simulink model "RL_fault_tolerance_simulation"  (R2024b)
settings: Solver=FixedStepAuto  StartTime=0.0  StopTime=500  FixedStep=0.1  RelTol=1e-3
PostLoadFcn:
  | RL_fault_tolerance_Setup
values from neighbouring files (symbols this model uses):
  D_default = 10    [rl_tolernace.m]
  t_gap = 1.4    [rl_tolernace.m]
  Ts = 0.1    [rl_tolernace.m]
  v_set = 28    [rl_tolernace.m]
undefined symbols (not defined in the file or in its folder): DiscIntNeverNeededParam, driving, egoID, lr, m, matlabshared, posSelector, R, tau
libraries: simulink x5, drivingscenarioandsensors x3, drivinglib x2, trackingutilitieslib x1, rllib x1, autolibshared x1
settings Model: SnapshotInterval=5  Creator=The MathWorks, Inc.  LastModifiedBy=user
settings SolverCC: AlgebraicLoopSolver=TrustRegion  MinimalZcImpactIntegration=on
settings OptimizationCC: DefaultParameterBehavior=Inlined  InlineInvariantSignals=on  ReuseModelBlockBuffer=off  PassReuseOutputArgsAs=Individual arguments  ZeroExternalMemoryAtStartup=off  OptimizeBlockOrder=speed  EfficientTunableParamExpr=on
settings DebuggingCC: ParameterTunabilityLossMsg=error  UnconnectedInputMsg=warning  UnconnectedOutputMsg=warning  UnconnectedLineMsg=warning  PregeneratedLibrarySubsystemCodeDiagnostic=none  ArithmeticOperatorsInVariantConditions=warning
settings HardwareCC: ProdLongLongMode=on
settings ModelReferenceCC: EnableRefExpFcnMdlSchedulingChecks=on  ModelReferenceNumInstancesAllowed=Single  PropagateVarSize=Only when enabling
settings SFSimCC: SimUseLocalCustomCode=off  CustomCodeUndefinedFunction=UseInterfaceOnly
settings RTWCC: Description=Embedded Coder  SystemTargetFile=ert.tlc  TemplateMakefile=ert_default_tmf  GenerateReport=on  RTWUseLocalCustomCode=off  BuildConfiguration=Faster Runs  IncludeHyperlinkInReport=on  LaunchReport=on  GenerateTraceInfo=on  GenerateTraceReport=on  GenerateTraceReportSl=on  GenerateTraceReportSf=on  GenerateTraceReportEml=on  GenerateCodeMetricsReport=on  GPUComputeCapability=3.5  DLArmComputeVersion=19.05
settings CodeAppCC: ForceParamTrailComments=on  IgnoreCustomStorageClasses=off  OperatorAnnotations=on  SimulinkDataObjDesc=on  SFDataObjDesc=on  CustomSymbolStrFcn=$N$M$F  InsertBlockDesc=on
settings ERTTargetCC: TargetLangStandard=C99 (ISO)  GenerateSampleERTMain=on  CombineSignalStateStructs=on  SuppressErrorStatus=on  RootIOFormat=Structure reference  RTWCAPISignals=on  ERTCustomFileTemplate=example_file_process.tlc  DynamicArrayContainerType=coder::array

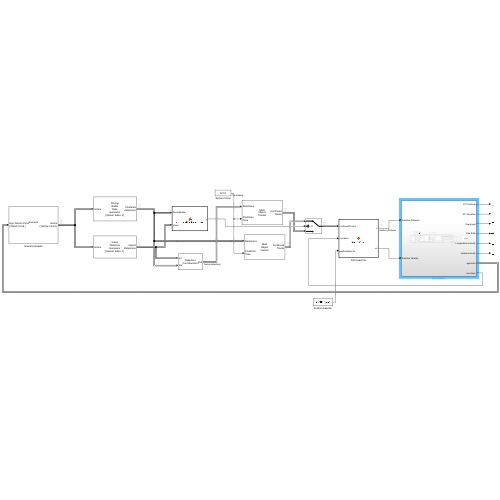
[thumbnail: Simulink's stored preview of the top-level diagram]
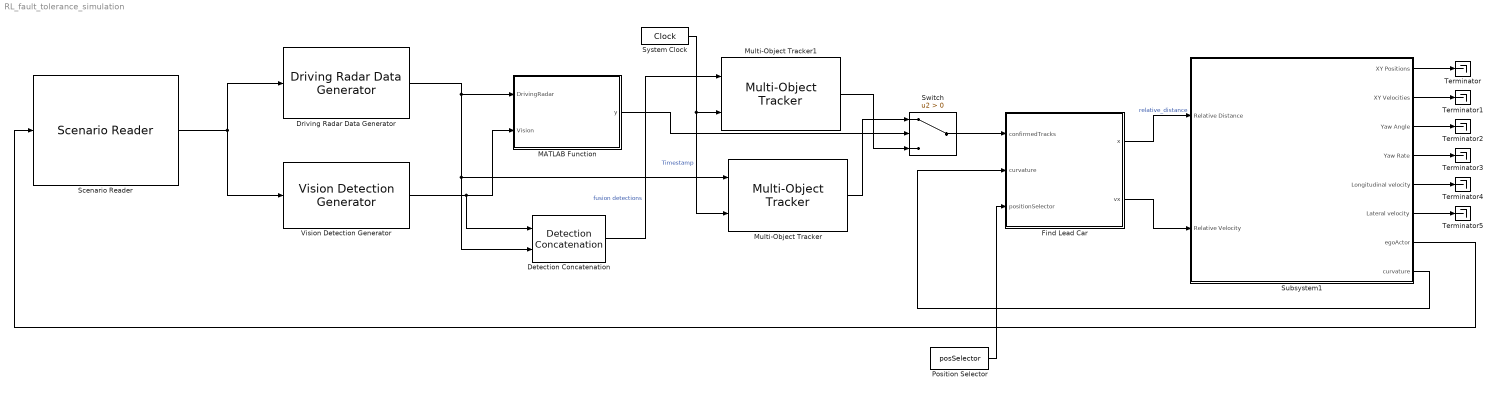
== system RL_fault_tolerance_simulation ==
  Detection Concatenation : trackingutilitieslib/Detection Concatenation  NumInputs=2  BusNameSource=Property  BusName=BusDetectionConcatenation  SimulateUsing=Interpreted execution
  Driving Radar Data Generator : drivingscenarioandsensors/Driving Radar Data Generator  SensorIndex=2  UpdateRate=10  MountingLocation=[ 3.7, 0, 0.2 ]  MountingAngles=[0 0 0]  HasElevation=off  HasRangeRate=on  HasNoise=on  HasFalseAlarms=on  HasOcclusion=on  MaxNumReportsSource=Property  MaxNumReports=50  TargetReportFormat=Clustered detections  DetectionCoordinates=Body  TrackCoordinates=Body  BusNameSource=Property  BusName=BusRadar  SimulateUsing=Interpreted execution  AzimuthResolution=4  ElevationResolution=5  RangeResolution=2.5  RangeRateResolution=0.5  AzimuthBiasFraction=0.1  ElevationBiasFraction=0.1  RangeBiasFraction=0.05  RangeRateBiasFraction=0.05  FieldOfView=[ 20, 5 ]  RangeLimits=[ 0, 174 ]  RangeRateLimits=[ -100, 100 ]  DetectionProbability=0.9  FalseAlarmRate=1e-06  ReferenceRange=100  ReferenceRCS=0  CenterFrequency=77e9  FilterInitializationFcn=initcvekf  ConfirmationThreshold=[2 3]  DeletionThreshold=[5 5]  InitialSeedSource=Repeatable  InitialSeed=0  UsedSeed=matlabshared.tracking.internal.SimulinkUtilities.seedManager(gcb)  ProfilesSource=Parameters  ProfilesParameters=driving.internal.ActorProfilesRadarParameters  ProfilesExpression=struct('ClassID',0,'Length',4.7,'Width',1.8,'Height',1.4,'OriginOffset',[-1.35 0 0],'RCSPattern',[10 10;10 10],'RCSAzimuthAngles',[-180 180],'RCSElevationAngles',[-90 90])
  Find Lead Car : MATLAB Function  TreatAsAtomicUnit=on
  MATLAB Function : MATLAB Function  TreatAsAtomicUnit=on
  Multi-Object Tracker : drivinglib/Multi-Object Tracker  TrackerIndex=uint32( 0 )  FilterInitializationFcn=initcvekf  AssignmentThreshold=assigThresh  ConfirmationThreshold=[ 2, 3 ]  DeletionThreshold=[ 5, 5 ]  MaxNumTracks=numTracks  MaxNumSensors=numSensors  OOSMHandling=Terminate  StateParametersSimulink=struct  HasStateParametersInput=off  TimeInputSource=Input port  HasCostMatrixInput=off  HasDetectableTrackIDsInput=off  BusNameSource=Property  BusName=BusMultiObjectTracker  TentativeTracksOutputPort=off  AllTracksOutputPort=off  SimulateUsing=Interpreted execution
  Multi-Object Tracker1 : drivinglib/Multi-Object Tracker  TrackerIndex=uint32( 0 )  FilterInitializationFcn=initcvekf  AssignmentThreshold=assigThresh  ConfirmationThreshold=[ 2, 3 ]  DeletionThreshold=[ 5, 5 ]  MaxNumTracks=numTracks  MaxNumSensors=numSensors  OOSMHandling=Terminate  StateParametersSimulink=struct  HasStateParametersInput=off  TimeInputSource=Input port  HasCostMatrixInput=off  HasDetectableTrackIDsInput=off  BusNameSource=Property  BusName=BusMultiObjectTracker  TentativeTracksOutputPort=off  AllTracksOutputPort=off  SimulateUsing=Interpreted execution
  Position Selector : Constant  Value=posSelector
  Scenario Reader : drivingscenarioandsensors/Scenario Reader  ScenarioSource=From workspace  ScenarioFileName=ACCTestBenchScenario.mat  ScenarioVariableName=scenario  OutputCoordinateSystem=Vehicle coordinates  EgoVehicleSource=Input port  EgoVehicleActorID=egoID  OrientVehiclesOnRoad=off  OutputEgoVehiclePose=off  OutputEgoVehicleState=off  SampleTime=0.1  LaneBoundaryOutput=None  LaneBoundaryDistance=0:0.5:9.5  LaneBoundaryLocation=Center of lane markings  BusNameSource=Property  BusName=BusActors  BusNumActorsSource=Scenario  BusNumActors=100  BusName2Source=Auto  BusName2=BusLaneBoundaries  BusNumLaneBoundariesSource=Scenario  BusNumLaneBoundaries=10  BusName3Source=Auto  BusName3=BusEgoActor  BusName4Source=Auto  BusName4=BusEgoState  ShowCoordinateLabels=on  SimulateUsing=Interpreted execution
  Subsystem1 : Subsystem
  Switch : Switch  Criteria=u2 > Threshold  SaturateOnIntegerOverflow=off  InputSameDT=off
  System Clock : DigitalClock  SampleTime=Ts
  Terminator{,1..5} (6 alike) : Terminator
  Vision Detection Generator : drivingscenarioandsensors/Vision Detection Generator  SensorIndex=1  DetectorOutput=Objects only  UpdateInterval=0.1  LaneUpdateInterval=0.1  SensorLocation=[ 2.1, 0 ]  Height=1.1  Yaw=0  Pitch=1  Roll=0  BusNameSource=Property  BusName=BusVision  BusName2Source=Auto  BusName2=BusLaneDetections  MaxNumDetectionsSource=Property  MaxNumDetections=20  MaxNumLanesSource=Property  MaxNumLanes=30  DetectionCoordinates=Ego Cartesian  SimulateUsing=Interpreted execution  MaxRange=150  BoundingBoxAccuracy=5  ProcessNoiseIntensity=5  MaxSpeed=50  MaxAllowedOcclusion=0.5  MinObjectImageSize=[ 15, 15 ]  DetectionProbability=0.9  FalsePositivesPerImage=0.1  MinLaneImageSize=[ 20, 5 ]  LaneBoundaryAccuracy=3  HasNoise=on  InitialSeedSource=Repeatable  InitialSeed=0  UsedSeed=driving.internal.SimulinkUtilities.seedManager(gcb)  ActorProfilesSource=Parameters  ActorProfilesParameters=driving.internal.ActorProfilesParameters  ActorProfilesExpression=struct( 'ClassID', 0, 'Length', 4.7, 'Width', 1.8, 'Height', 1.4, 'OriginOffset', [ -1.35, 0, 0 ] )  Intrinsics=driving.internal.cameraIntrinsics
  wires:
  Subsystem1/1(XY Positions) -> Terminator/1
  Subsystem1/2(XY Velocities) -> Terminator1/1
  Subsystem1/3(Yaw Angle) -> Terminator2/1
  Subsystem1/4(Yaw Rate) -> Terminator3/1
  Subsystem1/5(Longitudinal velocity) -> Terminator4/1
  Subsystem1/6(Lateral velocity) -> Terminator5/1
  Find Lead Car/2(vx) -> Subsystem1/2(Relative Velocity)
  Find Lead Car/1(x) -> Subsystem1/1(Relative Distance)  "relative_distance"
  Subsystem1/8(curvature) -> Find Lead Car/2(curvature)
  Multi-Object Tracker/1 -> Switch/1
  System Clock/1 -> Multi-Object Tracker1/2, Multi-Object Tracker/2  "Timestamp"
  Position Selector/1 -> Find Lead Car/3(positionSelector)
  Subsystem1/7(egoActor) -> Scenario Reader/1
  Detection Concatenation/1 -> Multi-Object Tracker1/1  "fusion detections"
  Switch/1 -> Find Lead Car/1(confirmedTracks)
  Driving Radar Data Generator/1 -> Multi-Object Tracker/1, Detection Concatenation/2, MATLAB Function/1(DrivingRadar)
  Scenario Reader/1 -> Driving Radar Data Generator/1, Vision Detection Generator/1
  Vision Detection Generator/1 -> MATLAB Function/2(Vision), Detection Concatenation/1
  MATLAB Function/1(y) -> Switch/2
  Multi-Object Tracker1/1 -> Switch/3

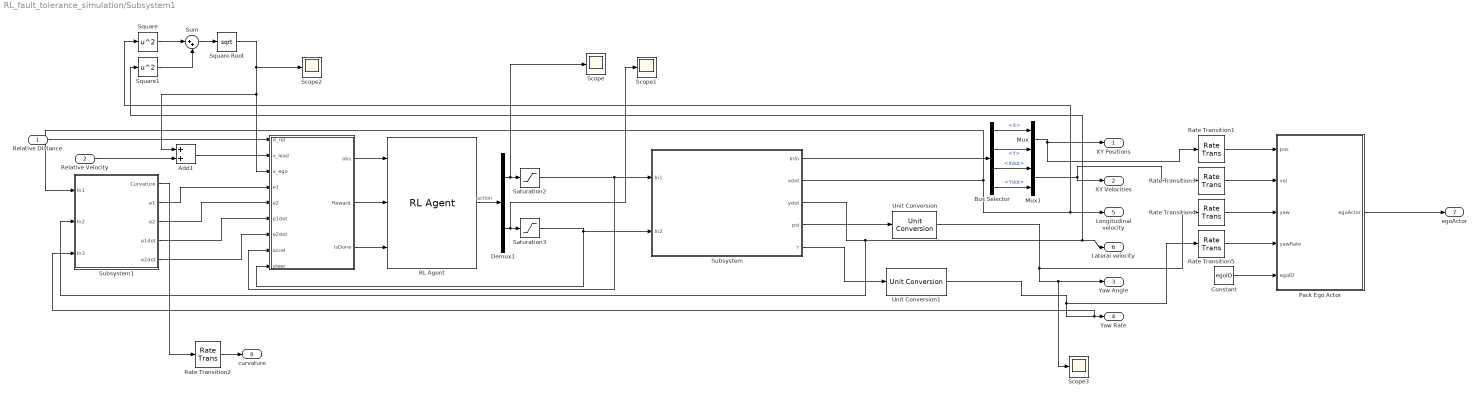
== system RL_fault_tolerance_simulation/Subsystem1 ==
  Relative Distance : Inport
  Relative Velocity : Inport  Port=2
  " " : Subsystem
  Add1 : Sum
  Bus Selector : BusSelector  OutputSignals=InertFrm.FrntAxl.Disp.X,InertFrm.FrntAxl.Disp.Y,InertFrm.FrntAxl.Vel.Xdot,InertFrm.FrntAxl.Vel.Ydot
  Constant : Constant  Value=egoID
  Demux1 : Demux  Outputs=2
  Mux : Mux  Inputs=2
  Mux1 : Mux  Inputs=2
  Pack Ego Actor : MATLAB Function  TreatAsAtomicUnit=on
  RL Agent : rllib/RL Agent  Agent=agent  ExternalActionAsInput=off  ProvideLastAction=off  ProvideCumRwd=off  TreatAsDirectFeedthrough=on  UseStrictObservationDataTypes=off
  Rate Transition{1..5} (5 alike) : RateTransition  OutPortSampleTime=Ts
  Saturation2 : Saturate  UpperLimit=2  LowerLimit=-3
  Saturation3 : Saturate  UpperLimit=0.1  LowerLimit=-0.1
  Scope{,1..3} (4 alike) : Scope
  Square : Math  Operator=square
  Square Root : Sqrt
  Square1 : Math  Operator=square
  Subsystem : Subsystem
  Subsystem1 : Subsystem
  Sum : Sum  Inputs=|++
  Unit Conversion : UnitConversion
  Unit Conversion1 : UnitConversion
  XY Positions : Outport  Unit=m  VectorParamsAs1DForOutWhenUnconnected=off
  XY Velocities : Outport  Port=2  Unit=m/s  VectorParamsAs1DForOutWhenUnconnected=off
  Yaw Angle : Outport  Port=3  Unit=deg  VectorParamsAs1DForOutWhenUnconnected=off
  Yaw Rate : Outport  Port=4  Unit=degree/s  VectorParamsAs1DForOutWhenUnconnected=off
  Longitudinal velocity : Outport  Port=5  VectorParamsAs1DForOutWhenUnconnected=off
  Lateral velocity : Outport  Port=6  VectorParamsAs1DForOutWhenUnconnected=off
  egoActor : Outport  Port=7
  curvature : Outport  Port=8
  wires:
  Bus Selector/4 -> Mux1/2  "<Ydot>"
  Mux1/1 -> XY Velocities/1, Rate Transition3/1
  Rate Transition2/1 -> curvature/1
  Saturation3/1 -> " "/9(steer), Subsystem/2(In2)
  " "/3(isDone) -> RL Agent/3
  Pack Ego Actor/1(egoActor) -> egoActor/1
  Mux/1 -> Rate Transition1/1, XY Positions/1
  " "/1(obs) -> RL Agent/1
  Constant/1 -> Pack Ego Actor/5(egoID)
  Saturation2/1 -> Subsystem/1(In1), " "/8(accel)
  Demux1/2 -> Scope1/1, Saturation3/1
  Unit Conversion1/1 -> Subsystem1/3(In3), Yaw Rate/1, Rate Transition5/1
  Relative Velocity/1 -> Add1/2
  Demux1/1 -> Scope/1, Saturation2/1
  Bus Selector/3 -> Mux1/1  "<Xdot>"
  Relative Distance/1 -> " "/1(d_rel)
  Rate Transition3/1 -> Pack Ego Actor/2(vel)
  Rate Transition5/1 -> Pack Ego Actor/4(yawRate)
  Rate Transition4/1 -> Pack Ego Actor/3(yaw)
  " "/2(Reward) -> RL Agent/2
  Rate Transition1/1 -> Pack Ego Actor/1(pos)
  Add1/1 -> " "/2(v_lead)
  Bus Selector/2 -> Mux/2  "<Y>"
  Bus Selector/1 -> Mux/1  "<X>"
  Unit Conversion/1 -> Scope3/1, Yaw Angle/1, Rate Transition4/1
  RL Agent/1 -> Demux1/1  "action"
  Subsystem/3(ydot) -> Lateral velocity/1, Square1/1, Subsystem1/2(In2)
  Subsystem/2(xdot) -> Longitudinal velocity/1, Square/1, Subsystem1/1(In1)
  Subsystem/1(Info) -> Bus Selector/1
  Subsystem/4(psi) -> Unit Conversion/1
  Subsystem/5(r) -> Unit Conversion1/1
  Subsystem1/1(Curvature) -> Rate Transition2/1
  Subsystem1/2(e1) -> " "/4(e1)
  Subsystem1/3(e2) -> " "/5(e2)
  Subsystem1/4(e1dot) -> " "/6(e1dot)
  Subsystem1/5(e2dot) -> " "/7(e2dot)
  Square/1 -> Sum/1
  Square1/1 -> Sum/2
  Sum/1 -> Square Root/1
  Square Root/1 -> " "/3(v_ego), Add1/1, Scope2/1

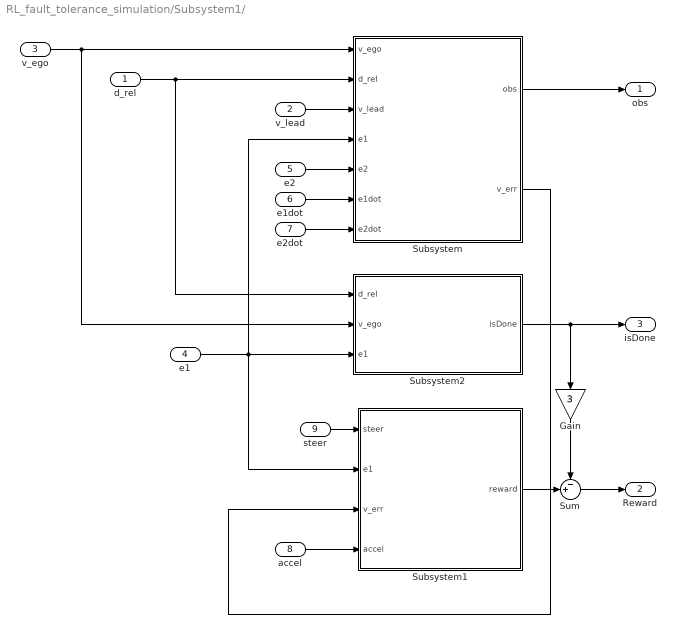
== system RL_fault_tolerance_simulation/Subsystem1/  ==
  d_rel : Inport
  v_lead : Inport  Port=2
  v_ego : Inport  Port=3
  e1 : Inport  Port=4
  e2 : Inport  Port=5
  e1dot : Inport  Port=6
  e2dot : Inport  Port=7
  accel : Inport  Port=8
  steer : Inport  Port=9
  Gain : Gain  Gain=3
  Subsystem : Subsystem
  Subsystem1 : Subsystem
  Subsystem2 : Subsystem
  Sum : Sum  Inputs=-+|
  obs : Outport  VectorParamsAs1DForOutWhenUnconnected=off
  Reward : Outport  Port=2  VectorParamsAs1DForOutWhenUnconnected=off
  isDone : Outport  Port=3  VectorParamsAs1DForOutWhenUnconnected=off
  wires:
  e2dot/1 -> Subsystem/7(e2dot)
  e1/1 -> Subsystem/4(e1), Subsystem2/3(e1), Subsystem1/2(e1)
  e2/1 -> Subsystem/5(e2)
  v_ego/1 -> Subsystem2/2(v_ego), Subsystem/1(v_ego)
  accel/1 -> Subsystem1/4(accel)
  Subsystem2/1(isDone) -> isDone/1, Gain/1
  Subsystem/2(v_err) -> Subsystem1/3(v_err)
  v_lead/1 -> Subsystem/3(v_lead)
  d_rel/1 -> Subsystem2/1(d_rel), Subsystem/2(d_rel)
  steer/1 -> Subsystem1/1(steer)
  Subsystem/1(obs) -> obs/1
  e1dot/1 -> Subsystem/6(e1dot)
  Subsystem1/1(reward) -> Sum/2
  Sum/1 -> Reward/1
  Gain/1 -> Sum/1

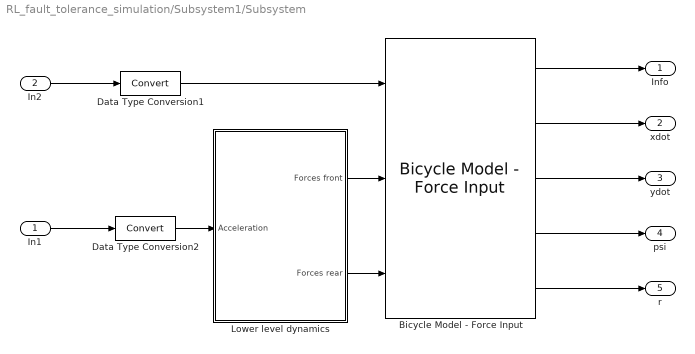
== system RL_fault_tolerance_simulation/Subsystem1/Subsystem ==
  In1 : Inport
  In2 : Inport  Port=2
  Bicycle Model - Force Input : autolibshared/Bicycle Model - Force Input  trackMode=Single (bicycle)  inputMode=External longitudinal forces  frontSteerMode=on  rearSteerMode=off  windMode=off  muMode=off  extFMode=off  extMMode=off  aMode=3  NF=2  NR=2  m=m  a=lf  b=lr  h=0.35  X_o=x0_ego  xdot_o=v0_ego  CalphaMode=off  sigmaMode=on  w=[1.4,1.4]  Cy_f=Cf  Cy_r=Cr  sigma_f=.1  sigma_r=.1  alpha_f_brk=[-.1 .1]  Cy_f_data=[-9e3 9e3]  alpha_r_brk=[-.1 .1]  Cy_r_data=[-9e3 9e3]  Y_o=y0_ego  ydot_o=0  Izz=Iz  psi_o=0  r_o=0  Af=0  Cd=.3  Cl=.1  Cpm=.1  beta_w=[0:0.01:0.3]  Cs=[0:0.03:0.9]  Cym=[0:0.01:0.3]  Pabs=101325  Tair=273  g=9.81  mu=1  xdot_tol=.01  Fznom=5000  Fxtire_sat=1e6  Fytire_sat=1e6  longOff=0  latOff=0  vertOff=0
      settings: LibrarySourceBlock=drivingscenarioandsensors/Bicycle Model - Force Input
  Data Type Conversion1 : DataTypeConversion  SaturateOnIntegerOverflow=off  RndMeth=Floor
  Data Type Conversion2 : DataTypeConversion  SaturateOnIntegerOverflow=off  RndMeth=Floor
  Lower level dynamics : Subsystem
  Info : Outport
  xdot : Outport  Port=2
  ydot : Outport  Port=3
  psi : Outport  Port=4
  r : Outport  Port=5
  wires:
  In1/1 -> Data Type Conversion2/1
  Bicycle Model - Force Input/3 -> ydot/1
  Lower level dynamics/2(Forces rear) -> Bicycle Model - Force Input/3
  Data Type Conversion1/1 -> Bicycle Model - Force Input/1
  Data Type Conversion2/1 -> Lower level dynamics/1(Acceleration)
  Lower level dynamics/1(Forces front) -> Bicycle Model - Force Input/2
  Bicycle Model - Force Input/4 -> psi/1
  Bicycle Model - Force Input/1 -> Info/1
  In2/1 -> Data Type Conversion1/1
  Bicycle Model - Force Input/2 -> xdot/1
  Bicycle Model - Force Input/5 -> r/1

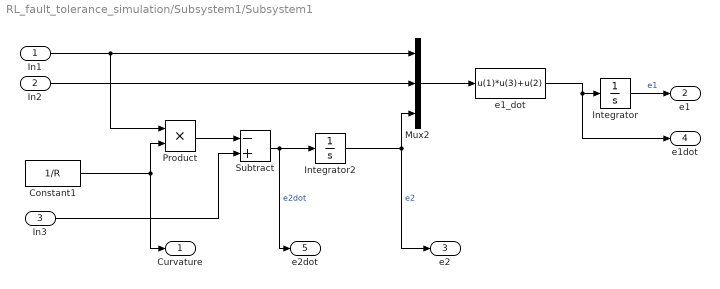
== system RL_fault_tolerance_simulation/Subsystem1/Subsystem1 ==
  In1 : Inport
  In2 : Inport  Port=2
  In3 : Inport  Port=3
  Constant1 : Constant  Value=1/R
  Integrator : Integrator  InitialCondition=0.2
  Integrator2 : Integrator  InitialCondition=-0.1
  Mux2 : Mux  Inputs=[1 1 1]
  Product : Product
  Subtract : Sum  Inputs=-+
  e1_dot : Fcn  Expr=u(1)*u(3)+u(2)
  Curvature : Outport
  e1 : Outport  Port=2
  e2 : Outport  Port=3
  e1dot : Outport  Port=4
  e2dot : Outport  Port=5
  wires:
  Integrator/1 -> e1/1  "e1"
  Constant1/1 -> Product/2, Curvature/1
  Product/1 -> Subtract/1
  In2/1 -> Mux2/2
  In1/1 -> Mux2/1, Product/1
  e1_dot/1 -> e1dot/1, Integrator/1
  Subtract/1 -> Integrator2/1, e2dot/1  "e2dot"
  Integrator2/1 -> e2/1, Mux2/3  "e2"
  Mux2/1 -> e1_dot/1
  In3/1 -> Subtract/2

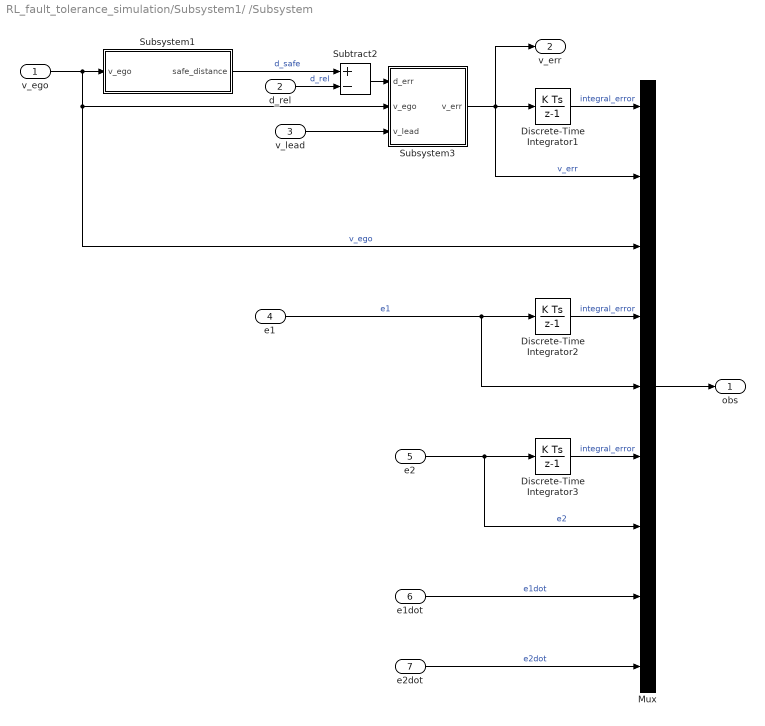
== system RL_fault_tolerance_simulation/Subsystem1/ /Subsystem ==
  v_ego : Inport
  d_rel : Inport  Port=2
  v_lead : Inport  Port=3
  e1 : Inport  Port=4
  e2 : Inport  Port=5
  e1dot : Inport  Port=6
  e2dot : Inport  Port=7
  Discrete-Time Integrator1 : DiscreteIntegrator  SampleTime=-1  ICPrevOutput=DiscIntNeverNeededParam  ICPrevScaledInput=DiscIntNeverNeededParam
  Discrete-Time Integrator2 : DiscreteIntegrator  SampleTime=-1  ICPrevOutput=DiscIntNeverNeededParam  ICPrevScaledInput=DiscIntNeverNeededParam
  Discrete-Time Integrator3 : DiscreteIntegrator  SampleTime=-1  ICPrevOutput=DiscIntNeverNeededParam  ICPrevScaledInput=DiscIntNeverNeededParam
  Mux : Mux  Inputs=9
  Subsystem1 : Subsystem
  Subsystem3 : Subsystem
  Subtract2 : Sum  Inputs=+-
  obs : Outport  VectorParamsAs1DForOutWhenUnconnected=off
  v_err : Outport  Port=2  VectorParamsAs1DForOutWhenUnconnected=off
  wires:
  v_lead/1 -> Subsystem3/3(v_lead)
  Subsystem3/1(v_err) -> v_err/1, Mux/2, Discrete-Time Integrator1/1  "v_err"
  Discrete-Time Integrator3/1 -> Mux/6  "integral_error"
  v_ego/1 -> Mux/3, Subsystem3/2(v_ego), Subsystem1/1(v_ego)  "v_ego"
  d_rel/1 -> Subtract2/2  "d_rel"
  e1/1 -> Mux/5, Discrete-Time Integrator2/1  "e1"
  Subsystem1/1(safe_distance) -> Subtract2/1  "d_safe"
  Discrete-Time Integrator1/1 -> Mux/1  "integral_error"
  e2/1 -> Mux/7, Discrete-Time Integrator3/1  "e2"
  Discrete-Time Integrator2/1 -> Mux/4  "integral_error"
  Mux/1 -> obs/1
  e1dot/1 -> Mux/8  "e1dot"
  e2dot/1 -> Mux/9  "e2dot"
  Subtract2/1 -> Subsystem3/1(d_err)

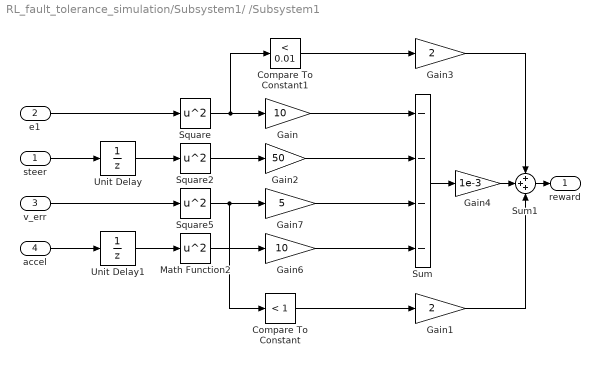
== system RL_fault_tolerance_simulation/Subsystem1/ /Subsystem1 ==
  steer : Inport
  e1 : Inport  Port=2
  v_err : Inport  Port=3
  accel : Inport  Port=4
  Compare To Constant : simulink/Logic and Bit Operations/Compare To Constant  relop=<  const=1  OutDataTypeStr=boolean
  Compare To Constant1 : simulink/Logic and Bit Operations/Compare To Constant  relop=<  const=0.01  OutDataTypeStr=boolean
  Gain : Gain  Gain=10
  Gain1 : Gain  Gain=2
  Gain2 : Gain  Gain=50
  Gain3 : Gain  Gain=2
  Gain4 : Gain  Gain=1e-3
  Gain6 : Gain  Gain=10
  Gain7 : Gain  Gain=5
  Math Function2 : Math  Operator=square  SignedPower=on
  Square : Math  Operator=square  SignedPower=on
  Square2 : Math  Operator=square  SignedPower=on
  Square5 : Math  Operator=square  SignedPower=on
  Sum : Sum  Inputs=----
  Sum1 : Sum  Inputs=+++
  Unit Delay : UnitDelay  SampleTime=-1  HasFrameUpgradeWarning=on
  Unit Delay1 : UnitDelay  SampleTime=-1  HasFrameUpgradeWarning=on
  reward : Outport  VectorParamsAs1DForOutWhenUnconnected=off
  wires:
  e1/1 -> Square/1
  Gain/1 -> Sum/1
  Square/1 -> Compare To Constant1/1, Gain/1
  steer/1 -> Unit Delay/1
  Square2/1 -> Gain2/1
  Unit Delay/1 -> Square2/1
  accel/1 -> Unit Delay1/1
  Unit Delay1/1 -> Math Function2/1
  Square5/1 -> Compare To Constant/1, Gain7/1
  Math Function2/1 -> Gain6/1
  Gain7/1 -> Sum/3
  v_err/1 -> Square5/1
  Gain6/1 -> Sum/4
  Gain2/1 -> Sum/2
  Sum1/1 -> reward/1
  Compare To Constant/1 -> Gain1/1
  Gain1/1 -> Sum1/3
  Compare To Constant1/1 -> Gain3/1
  Gain3/1 -> Sum1/1
  Sum/1 -> Gain4/1
  Gain4/1 -> Sum1/2

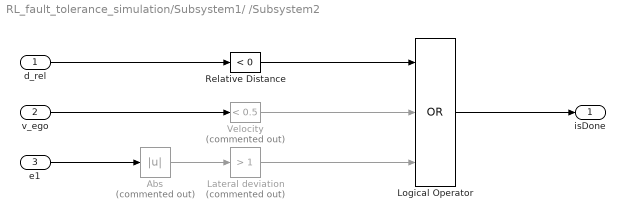
== system RL_fault_tolerance_simulation/Subsystem1/ /Subsystem2 ==
  d_rel : Inport
  v_ego : Inport  Port=2
  e1 : Inport  Port=3
  Abs : Abs  Commented=on  SaturateOnIntegerOverflow=off
  Lateral deviation : simulink/Logic and Bit Operations/Compare To Constant  Commented=on  relop=>  const=1  OutDataTypeStr=boolean
  Logical Operator : Logic  Operator=OR  Inputs=3  AllPortsSameDT=off  OutDataTypeStr=boolean
  Relative Distance : simulink/Logic and Bit Operations/Compare To Constant  relop=<  const=0  OutDataTypeStr=boolean
  Velocity : simulink/Logic and Bit Operations/Compare To Constant  Commented=on  relop=<  const=0.5  OutDataTypeStr=boolean
  isDone : Outport  VectorParamsAs1DForOutWhenUnconnected=off
  wires:
  Velocity/1 -> Logical Operator/2
  Relative Distance/1 -> Logical Operator/1
  d_rel/1 -> Relative Distance/1
  Logical Operator/1 -> isDone/1
  v_ego/1 -> Velocity/1
  Abs/1 -> Lateral deviation/1
  Lateral deviation/1 -> Logical Operator/3
  e1/1 -> Abs/1

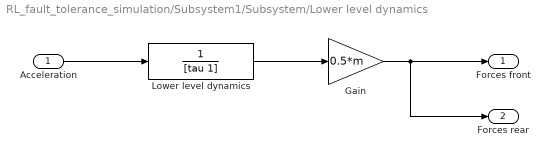
== system RL_fault_tolerance_simulation/Subsystem1/Subsystem/Lower level dynamics ==
  Acceleration : Inport
  Gain : Gain  Gain=0.5*m
  Lower level dynamics : TransferFcn  Denominator=[tau 1]
  Forces front : Outport  VectorParamsAs1DForOutWhenUnconnected=off
  Forces rear : Outport  Port=2  VectorParamsAs1DForOutWhenUnconnected=off
  wires:
  Gain/1 -> Forces rear/1, Forces front/1
  Acceleration/1 -> Lower level dynamics/1
  Lower level dynamics/1 -> Gain/1

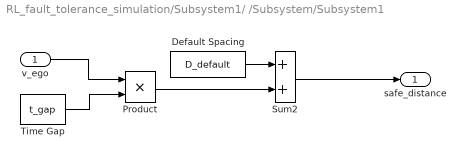
== system RL_fault_tolerance_simulation/Subsystem1/ /Subsystem/Subsystem1 ==
  v_ego : Inport
  Default Spacing : Constant  Value=D_default  SampleTime=Ts
  Product : Product
  Sum2 : Sum
  Time Gap : Constant  Value=t_gap  SampleTime=Ts
  safe_distance : Outport  VectorParamsAs1DForOutWhenUnconnected=off
  wires:
  v_ego/1 -> Product/1
  Default Spacing/1 -> Sum2/1
  Time Gap/1 -> Product/2
  Product/1 -> Sum2/2
  Sum2/1 -> safe_distance/1

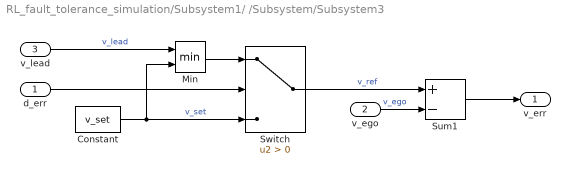
== system RL_fault_tolerance_simulation/Subsystem1/ /Subsystem/Subsystem3 ==
  d_err : Inport
  v_ego : Inport  Port=2
  v_lead : Inport  Port=3
  Constant : Constant  Value=v_set
  Min : MinMax  Inputs=2
  Sum1 : Sum  Inputs=+-
  Switch : Switch  Criteria=u2 > Threshold  SaturateOnIntegerOverflow=off  InputSameDT=off
  v_err : Outport  VectorParamsAs1DForOutWhenUnconnected=off
  wires:
  v_lead/1 -> Min/1  "v_lead"
  Min/1 -> Switch/1
  Constant/1 -> Switch/3, Min/2  "v_set"
  d_err/1 -> Switch/2
  Switch/1 -> Sum1/1  "v_ref"
  v_ego/1 -> Sum1/2  "v_ego"
  Sum1/1 -> v_err/1

== matlab function RL_fault_tolerance_simulation/MATLAB Function ==
  data: DrivingRadar input; y output; Vision input
function y = compareNumDetections(DrivingRadar, Vision) 
radarCnt  = double(DrivingRadar.NumDetections);
visionCnt = double(Vision.NumDetections);

if radarCnt > visionCnt
    y = uint8(1);
else
    y = uint8(0);
end
end

== matlab function RL_fault_tolerance_simulation/Find Lead Car ==
  data: confirmedTracks input; x output double size=[1 1]; vx output size=[1 1]; curvature input; positionSelector input
function [x,vx] = findLeadCar(confirmedTracks, curvature, positionSelector)

numStates = 6;
laneWidth = 3.6;
halfLaneWidth = laneWidth/2;
maxX = cast(1000, 'like', confirmedTracks.Tracks(1).State);
trackID = 0;
for i = 1:confirmedTracks.NumTracks
    position = positionSelector * confirmedTracks.Tracks(i).State;
    x = position(1);
    y = position(2);

    if x < maxX && x > 0
        yleftLane  = polyval([curvature/2, 0,  halfLaneWidth],x);
        yrightLane = polyval([curvature/2, 0, -halfLaneWidth],x);

        if (yrightLane <= y) && (y <= yleftLane)
            maxX = x;
            trackID = i;
        end
    end
end

if trackID>0
    mioState = confirmedTracks.Tracks(trackID).State;
else
    mioState = inf(numStates,1,'like',confirmedTracks.Tracks(1).State);
end

x = mioState(1);
vx = mioState(2);

== matlab function RL_fault_tolerance_simulation/Subsystem1/Pack Ego Actor ==
  data: pos input; egoActor output Bus: BusActorsActors size=1; vel input; yaw input; yawRate input; egoID input
function egoActor  = packEgo(pos,vel,yaw,yawRate,egoID)

egoActor = struct(...
    'ActorID',egoID,...
    'Position', [pos(1) pos(2) 0], ...
    'Velocity', [vel(1) vel(2) 0], ...
    'Roll', 0, ...
    'Pitch', 0, ...
    'Yaw', yaw, ...
    'AngularVelocity', [0 0 yawRate]);
